simulink model "Tank"  (R2020a)
settings: Solver=VariableStepAuto  StartTime=0.0  StopTime=200  RelTol=1e-3
values from neighbouring files (symbols this model uses):
  D = 4    [load_data.m]
  Pump = 2    [load_data.m]
settings Model: Creator=lydialagorga  LastModifiedBy=lydialagorga

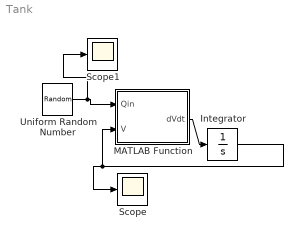
== system Tank ==
  Integrator : Integrator  LimitOutput=on  LowerSaturationLimit=0
  MATLAB Function : MATLAB Function  TreatAsAtomicUnit=on
  Scope : Scope
  Scope1 : Scope
  Uniform Random Number : UniformRandomNumber  Minimum=2  Maximum=8  SampleTime=1
  wires:
  Uniform Random Number/1 -> Scope1/1, MATLAB Function/1(Qin)
  MATLAB Function/1(dVdt) -> Integrator/1
  Integrator/1 -> Scope/1, MATLAB Function/2(V)

== matlab function Tank/MATLAB Function ==
  data: Qin input; dVdt output; V input; D parameter; Pump parameter
function dVdt = tank(Qin, V, D, Pump)
Qout = Pump;
if V > 220
    Qout = Qin;
end
%tankXA = pi*(4*D^2); %cross section area in m^2
%height = V/tankXA; %height of fluid in tank m
%pipe = 1/2 m
dVdt = Qin - Qout; % rate of change of tank volume
